simulink model "QCarCameraTest"  (R2021a)
settings: Solver=ode1  StartTime=0.0  StopTime=inf  FixedStep=1/30  RelTol=1e-3  EnableMultiTasking=on
undefined symbols (not defined in the file): Video3D
libraries: quarc_library x20
settings Model: ExtModeTrigDuration=10000  Creator=mbohra  LastModifiedBy=mbohra
settings SolverCC: AlgebraicLoopSolver=TrustRegion  PositivePriorityOrder=on
settings DataIOCC: ReturnWorkspaceOutputs=off
settings DebuggingCC: SFMachineParentedDataDiag=warning  ArithmeticOperatorsInVariantConditions=warning
settings SFSimCC: SimUseLocalCustomCode=off  CustomCodeUndefinedFunction=UseInterfaceOnly
settings RTWCC: Description=QUARC Win64 Target Using Toolchain  SystemTargetFile=quarc_win64.tlc  TemplateMakefile=quarc_default_tmf  RTWUseLocalCustomCode=off  Toolchain=QUARC win64 | nmake (64-bit Windows)  BuildConfiguration=Faster Runs
settings CodeAppCC: StateflowObjectComments=on
settings STFCustomTargetCC: TargetLangStandard=C99 (ISO)  ConcurrentExecutionCompliant=on  SystemTargetFile=quarc_win64.tlc
settings GRTTargetCC: ParMdlRefBuildCompliant=off  CompOptLevelCompliant=off  CombineOutputUpdateFcns=off  MatFileLogging=off  CPPClassGenCompliant=off  GRTInterface=on  ExtMode=on  ExtModeMexFile=quarc_comm
settings ConfigComp: CovMetricSettings=dswe

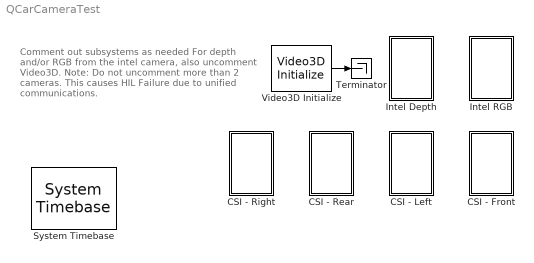
== system QCarCameraTest ==
  note: Comment out subsystems as needed
      |
      | For depth and/or RGB from the intel camera,
      | also uncomment Video3D.
      |
      | Note: Do not uncomment more than 2 cameras.
      | This causes HIL Failure due to
      | unified communications.
  CSI - Front : Subsystem
  CSI - Left : Subsystem
  CSI - Rear : Subsystem
  CSI - Right : Subsystem
  Intel Depth : Subsystem
  Intel RGB : Subsystem
  System Timebase : quarc_library/Advanced/Timing/System Timebase  stop_on_overrun=off
      settings: SourceProductName=QUARC Targets
  Terminator : Terminator
  Video3D Initialize : quarc_library/Multimedia/Video3D Initialize  object_name=Video3D-1  source=Device  identifier=0@tcpip://localhost:18965  file=sample.bag  sample_time=qc_get_step_size  active=on
  wires:
  Video3D Initialize/1 -> Terminator/1

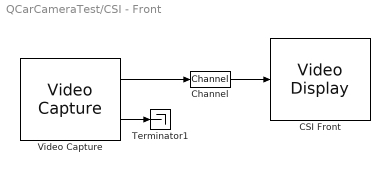
== system QCarCameraTest/CSI - Front ==
  CSI Front : quarc_library/Multimedia/Video Display  Tag=QCarCameraTest/CSI - Front/CSI Front  sample_time=-1  use_hardware=on
  Channel : quarc_library/Signal Routing/Channel  channel=0  buffer_size=1
  Terminator1 : Terminator
  Video Capture : quarc_library/Multimedia/Video Capture  source=device  device=3@tcpip://localhost:18964  filename=sample_movie.mov  value=[0 0; 0 0]  resolution=820 x 410  width=820  height=410  output_format=MATLAB RGB (HxWx3)  data_type=uint8  sample_time=qc_get_step_size  brightness_override=off  brightness=50.0  contrast_override=off  contrast=50.0  hue_override=off  hue=50.0  saturation_override=off  saturation=50.0  sharpness_override=off  sharpness=50.0  gamma_override=off  gamma=50.0  coloreffect_override=off  coloreffect=None  whitebalance_override=off  whitebalance=50.0  backlightcompensation_override=off  backlightcompensation=0.0  gain_override=off  gain=50.0  pan_override=off  pan=50.0  tilt_override=off  tilt=50.0  roll_override=off  roll=50.0  zoom_override=off  zoom=0.0  exposure_override=off  exposure=50.0  iris_override=off  iris=50.0  focus_override=off  focus=0.0
      settings: SourceProductName=QUARC Targets
  wires:
  Video Capture/2 -> Terminator1/1
  Video Capture/1 -> Channel/1
  Channel/1 -> CSI Front/1

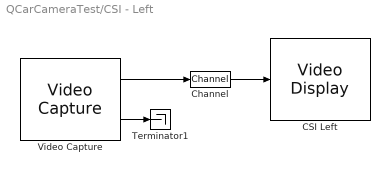
== system QCarCameraTest/CSI - Left ==
  CSI Left : quarc_library/Multimedia/Video Display  Tag=QCarCameraTest/CSI - Left/CSI Left  sample_time=-1  use_hardware=on
  Channel : quarc_library/Signal Routing/Channel  channel=1  buffer_size=1
  Terminator1 : Terminator
  Video Capture : quarc_library/Multimedia/Video Capture  source=device  device=2@tcpip://localhost:18963  filename=sample_movie.mov  value=[0 0; 0 0]  resolution=820 x 410  width=820  height=410  output_format=MATLAB RGB (HxWx3)  data_type=uint8  sample_time=qc_get_step_size  brightness_override=off  brightness=50.0  contrast_override=off  contrast=50.0  hue_override=off  hue=50.0  saturation_override=off  saturation=50.0  sharpness_override=off  sharpness=50.0  gamma_override=off  gamma=50.0  coloreffect_override=off  coloreffect=None  whitebalance_override=off  whitebalance=50.0  backlightcompensation_override=off  backlightcompensation=0.0  gain_override=off  gain=50.0  pan_override=off  pan=50.0  tilt_override=off  tilt=50.0  roll_override=off  roll=50.0  zoom_override=off  zoom=0.0  exposure_override=off  exposure=50.0  iris_override=off  iris=50.0  focus_override=off  focus=0.0
      settings: SourceProductName=QUARC Targets
  wires:
  Channel/1 -> CSI Left/1
  Video Capture/1 -> Channel/1
  Video Capture/2 -> Terminator1/1

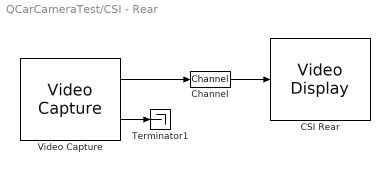
== system QCarCameraTest/CSI - Rear ==
  CSI Rear : quarc_library/Multimedia/Video Display  Tag=QCarCameraTest/CSI - Rear/CSI Rear  sample_time=-1  use_hardware=on
  Channel : quarc_library/Signal Routing/Channel  channel=2  buffer_size=1
  Terminator1 : Terminator
  Video Capture : quarc_library/Multimedia/Video Capture  source=device  device=1@tcpip://localhost:18962  filename=sample_movie.mov  value=[0 0; 0 0]  resolution=820 x 410  width=820  height=410  output_format=MATLAB RGB (HxWx3)  data_type=uint8  sample_time=qc_get_step_size  brightness_override=off  brightness=50.0  contrast_override=off  contrast=50.0  hue_override=off  hue=50.0  saturation_override=off  saturation=50.0  sharpness_override=off  sharpness=50.0  gamma_override=off  gamma=50.0  coloreffect_override=off  coloreffect=None  whitebalance_override=off  whitebalance=50.0  backlightcompensation_override=off  backlightcompensation=0.0  gain_override=off  gain=50.0  pan_override=off  pan=50.0  tilt_override=off  tilt=50.0  roll_override=off  roll=50.0  zoom_override=off  zoom=0.0  exposure_override=off  exposure=50.0  iris_override=off  iris=50.0  focus_override=off  focus=0.0
      settings: SourceProductName=QUARC Targets
  wires:
  Video Capture/2 -> Terminator1/1
  Video Capture/1 -> Channel/1
  Channel/1 -> CSI Rear/1

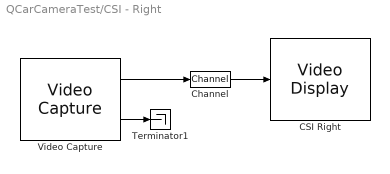
== system QCarCameraTest/CSI - Right ==
  CSI Right : quarc_library/Multimedia/Video Display  Tag=QCarCameraTest/CSI - Right/CSI Right  sample_time=-1  use_hardware=on
  Channel : quarc_library/Signal Routing/Channel  channel=3  buffer_size=1
  Terminator1 : Terminator
  Video Capture : quarc_library/Multimedia/Video Capture  source=device  device=0@tcpip://localhost:18961  filename=sample_movie.mov  value=[0 0; 0 0]  resolution=820 x 410  width=820  height=410  output_format=MATLAB RGB (HxWx3)  data_type=uint8  sample_time=qc_get_step_size  brightness_override=off  brightness=50.0  contrast_override=off  contrast=50.0  hue_override=off  hue=50.0  saturation_override=off  saturation=50.0  sharpness_override=off  sharpness=50.0  gamma_override=off  gamma=50.0  coloreffect_override=off  coloreffect=None  whitebalance_override=off  whitebalance=50.0  backlightcompensation_override=off  backlightcompensation=0.0  gain_override=off  gain=50.0  pan_override=off  pan=50.0  tilt_override=off  tilt=50.0  roll_override=off  roll=50.0  zoom_override=off  zoom=0.0  exposure_override=off  exposure=50.0  iris_override=off  iris=50.0  focus_override=off  focus=0.0
      settings: SourceProductName=QUARC Targets
  wires:
  Channel/1 -> CSI Right/1
  Video Capture/1 -> Channel/1
  Video Capture/2 -> Terminator1/1

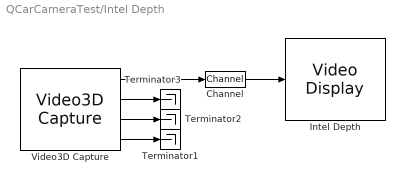
== system QCarCameraTest/Intel Depth ==
  Channel : quarc_library/Signal Routing/Channel  channel=4  buffer_size=1
  Intel Depth : quarc_library/Multimedia/Video Display  Tag=QCarCameraTest/Intel Depth/Intel Depth  sample_time=-1  use_hardware=on
  Terminator1 : Terminator
  Terminator2 : Terminator
  Terminator3 : Terminator
  Video3D Capture : quarc_library/Multimedia/Video3D Capture  object_name=Video3D-1  stream_type=Depth  stream_index=0  resolution=640 x 480  width=640  height=480  output_format=MATLAB greyscale (HxW)  data_type=uint8  sample_time=qc_get_step_size  camera_intrinsics=off  depth_scale=off  brightness_override=off  brightness=50.0  contrast_override=off  contrast=50.0  hue_override=off  hue=50.0  saturation_override=off  saturation=50.0  sharpness_override=off  sharpness=50.0  gamma_override=off  gamma=50.0  gain_override=off  gain=50.0  backlightcompensation_override=off  backlightcompensation=50.0  whitebalance_override=Automatic white balance  whitebalance=50.0  exposure_override=Automatic exposure  exposure=30.0  emitter=Enable laser emitter  preset=Do not set camera presets
  wires:
  Channel/1 -> Intel Depth/1
  Video3D Capture/1 -> Channel/1
  Video3D Capture/3 -> Terminator2/1
  Video3D Capture/4 -> Terminator1/1
  Video3D Capture/2 -> Terminator3/1

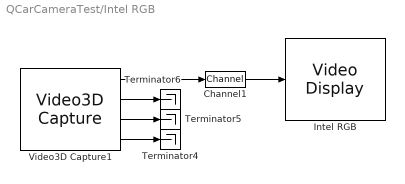
== system QCarCameraTest/Intel RGB ==
  Channel1 : quarc_library/Signal Routing/Channel  channel=5  buffer_size=1
  Intel RGB : quarc_library/Multimedia/Video Display  Tag=QCarCameraTest/Intel RGB/Intel RGB  sample_time=-1  use_hardware=on
  Terminator4 : Terminator
  Terminator5 : Terminator
  Terminator6 : Terminator
  Video3D Capture1 : quarc_library/Multimedia/Video3D Capture  object_name=Video3D-1  stream_type=RGB  stream_index=0  resolution=640 x 480  width=640  height=480  output_format=MATLAB RGB (HxWx3)  data_type=uint8  sample_time=qc_get_step_size  camera_intrinsics=off  depth_scale=off  brightness_override=off  brightness=50.0  contrast_override=off  contrast=50.0  hue_override=off  hue=50.0  saturation_override=off  saturation=50.0  sharpness_override=off  sharpness=50.0  gamma_override=off  gamma=50.0  gain_override=off  gain=50.0  backlightcompensation_override=off  backlightcompensation=50.0  whitebalance_override=Automatic white balance  whitebalance=50.0  exposure_override=Automatic exposure  exposure=30.0  emitter=Enable laser emitter  preset=Do not set camera presets
  wires:
  Video3D Capture1/2 -> Terminator6/1
  Video3D Capture1/4 -> Terminator4/1
  Video3D Capture1/1 -> Channel1/1
  Channel1/1 -> Intel RGB/1
  Video3D Capture1/3 -> Terminator5/1
